simulink model "IntegrityControlModule"  (R2020b)
settings: Solver=VariableStepAuto  StartTime=0.0  StopTime=10.0  RelTol=1e-3
settings Model: Creator=leonk  LastModifiedBy=leonk

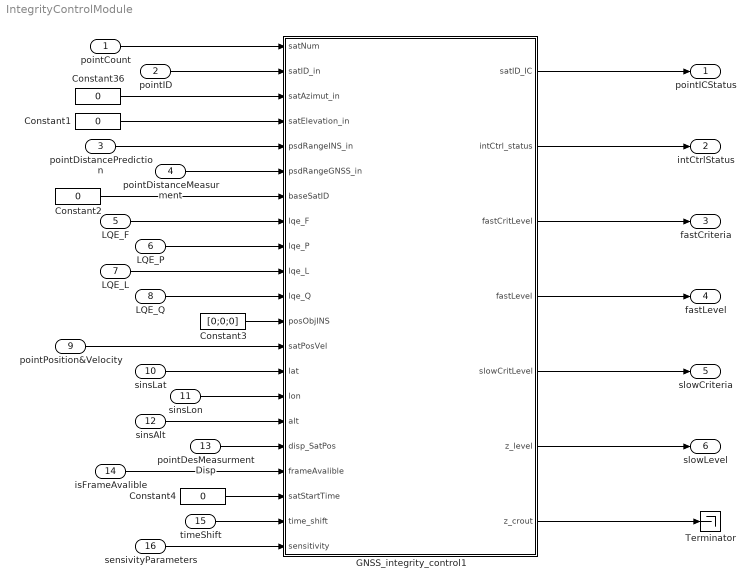
== system IntegrityControlModule ==
  pointCount : Inport  OutDataTypeStr=uint8
  pointID : Inport  Port=2
  pointDistancePrediction : Inport  Port=3  PortDimensions=[8,1]
  pointDistanceMeasurment : Inport  Port=4  PortDimensions=[8,1]
  LQE_F : Inport  Port=5
  LQE_P : Inport  Port=6
  LQE_L : Inport  Port=7
  LQE_Q : Inport  Port=8
  pointPosition&Velocity : Inport  Port=9  PortDimensions=[6,8]
  sinsLat : Inport  Port=10  PortDimensions=1
  sinsLon : Inport  Port=11  PortDimensions=1
  sinsAlt : Inport  Port=12  PortDimensions=1
  pointDesMeasurmentDisp : Inport  Port=13  PortDimensions=1
  isFrameAvalible : Inport  Port=14  OutDataTypeStr=uint8  PortDimensions=1
  timeShift : Inport  Port=15  PortDimensions=1
  sensivityParameters : Inport  Port=16  PortDimensions=[4,1]
  Constant{1..2,4,36} (4 alike) : Constant  Value=0
  Constant3 : Constant  Value=[0;0;0]
  GNSS_integrity_control1 : MATLAB Function  TreatAsAtomicUnit=on
  Terminator : Terminator
  pointICStatus : Outport  PortDimensions=32
  intCtrlStatus : Outport  Port=2  PortDimensions=32
  fastCriteria : Outport  Port=3
  fastLevel : Outport  Port=4  PortDimensions=32
  slowCriteria : Outport  Port=5  PortDimensions=32
  slowLevel : Outport  Port=6
  wires:
  pointCount/1 -> GNSS_integrity_control1/1(satNum)
  pointID/1 -> GNSS_integrity_control1/2(satID_in)
  Constant36/1 -> GNSS_integrity_control1/3(satAzimut_in)
  Constant1/1 -> GNSS_integrity_control1/4(satElevation_in)
  pointDistancePrediction/1 -> GNSS_integrity_control1/5(psdRangeINS_in)
  pointDistanceMeasurment/1 -> GNSS_integrity_control1/6(psdRangeGNSS_in)
  Constant2/1 -> GNSS_integrity_control1/7(baseSatID)
  LQE_F/1 -> GNSS_integrity_control1/8(lqe_F)
  LQE_P/1 -> GNSS_integrity_control1/9(lqe_P)
  LQE_L/1 -> GNSS_integrity_control1/10(lqe_L)
  LQE_Q/1 -> GNSS_integrity_control1/11(lqe_Q)
  Constant3/1 -> GNSS_integrity_control1/12(posObjINS)
  pointPosition&Velocity/1 -> GNSS_integrity_control1/13(satPosVel)
  sinsLat/1 -> GNSS_integrity_control1/14(lat)
  sinsLon/1 -> GNSS_integrity_control1/15(lon)
  sinsAlt/1 -> GNSS_integrity_control1/16(alt)
  isFrameAvalible/1 -> GNSS_integrity_control1/18(frameAvalible)
  Constant4/1 -> GNSS_integrity_control1/19(satStartTime)
  timeShift/1 -> GNSS_integrity_control1/20(time_shift)
  sensivityParameters/1 -> GNSS_integrity_control1/21(sensitivity)
  GNSS_integrity_control1/2(intCtrl_status) -> intCtrlStatus/1
  GNSS_integrity_control1/1(satID_IC) -> pointICStatus/1
  GNSS_integrity_control1/3(fastCritLevel) -> fastCriteria/1
  GNSS_integrity_control1/4(fastLevel) -> fastLevel/1
  GNSS_integrity_control1/5(slowCritLevel) -> slowCriteria/1
  GNSS_integrity_control1/6(z_level) -> slowLevel/1
  GNSS_integrity_control1/7(z_crout) -> Terminator/1
  pointDesMeasurmentDisp/1 -> GNSS_integrity_control1/17(disp_SatPos)

== matlab function IntegrityControlModule/GNSS_integrity_control1 ==
  data: satNum input uint8 size=1; satID_in input; satAzimut_in input; satElevation_in input; psdRangeINS_in input; psdRangeGNSS_in input; baseSatID input uint8 size=1; satID_IC output uint8; intCtrl_status output uint8 size=1; lqe_F input; lqe_P input; lqe_L input; lqe_Q input; posObjINS input size=3; satPosVel input; lat input; lon input; alt input; disp_SatPos input; frameAvalible input; fastCritLevel output; fastLevel output; slowCritLevel output; satStartTime input; time_shift input; sensitivity input size=[4,1]; z_level output; z_crout output

function [satID_IC, intCtrl_status, fastCritLevel, fastLevel, slowCritLevel,...
          z_level, z_crout]=  integrity_control(satNum, satID_in, satAzimut_in, satElevation_in, ...
                                                         psdRangeINS_in, psdRangeGNSS_in, baseSatID,...                                                     
                                                         lqe_F, lqe_P, lqe_L, lqe_Q, posObjINS, satPosVel, lat, lon, alt, disp_SatPos, frameAvalible, satStartTime, time_shift, sensitivity)

    persistent intCtrl qq time
%--------------------------------------------------------------------------
%Константы
    disp_SatVel = 0.03;
    
    
    
    if isempty(intCtrl)
               
        qq = 0;
        time = 0;
        slowWindow = 600;% set max for code generation
        satLimit   = 8;
        
%         intCtrl.sensitivity = zeros(3,1);
        intCtrl.slowSensitivity = sensitivity(3);
        
        intCtrl.fastInit = uint8(0);
        intCtrl.psdRangeFast = zeros(satLimit,3);
        intCtrl.fastSatList = zeros(satLimit,1);
        
        
        intCtrl.slowInit = uint8(0);
        intCtrl.psdRangeSlow = ones(slowWindow,satLimit);
        intCtrl.slowSatList  = zeros(satLimit,1);
        
        intCtrl.probSatID = uint8(zeros(satLimit,1));
        intCtrl.moniSatID = uint8(zeros(satLimit,1));
        
        intCtrl.probSatNum = uint8(0);
        intCtrl.moniSatNum = uint8(0);
        
        intCtrl.baseSatID = uint8(0);
        
        intCtrl.satLossFrame     = zeros(satLimit,2); %Строка 1 не задейстоввана?
        intCtrl.satLossFrameAlow = uint8(10);
        
        intCtrl.slowMean = zeros(satLimit,2);
        intCtrl.slowDisp = zeros(satLimit,1);
        
        intCtrl.fastExpt = zeros(satLimit,1);%Не задействовано
        
        intCtrl.fastExptCriteria = zeros(satLimit,2);
        
        intCtrl.criteriaScale = ones(2,1) .* [sensitivity(1); sensitivity(2)]; 
        
        intCtrl.slowWindow      = slowWindow;
        intCtrl.slowWindow_size = sensitivity(4);
        intCtrl.satLimit        = satLimit;
    end
%--------------------------------------------------------------------------
%Объявление выходых параметров 
    satID_IC       = uint8(zeros(8 ,1));%uint8(zeros(intCtrl.satLimit ,1));
    fastCritLevel  =       zeros(8,1);%zeros(intCtrl.satLimit ,1);
    fastLevel      =       zeros(8,1);%zeros(intCtrl.satLimit ,1);
    slowCritLevel  =       zeros(8,1);%zeros(intCtrl.satLimit ,1);
    intCtrl_status =       uint8(1); %%uint8(1); %
    z_crout        =       zeros(1,1);%zeros(1,1);
    z_level        =       zeros(8,1);%zeros(intCtrl.satLimit ,1);
    
%--------------------------------------------------------------------------
%Костыль для подержания много спутников (Если всегда +- 8 но подскакивает до 12)

    satID        = uint8(zeros(intCtrl.satLimit,1));
    satAzimut    =       zeros(intCtrl.satLimit,1);
    satElevation =       zeros(intCtrl.satLimit,1);
    psdRangeINS  =       zeros(intCtrl.satLimit,1);
    psdRangeGNSS =       zeros(intCtrl.satLimit,1);
    
    for ii = 1:satNum
        satID(ii)        = satID_in(ii);
        satAzimut(ii)    = satAzimut_in(ii);
        satElevation(ii) = satElevation_in(ii);
        psdRangeINS(ii)  = psdRangeINS_in(ii);
        psdRangeGNSS(ii) = psdRangeGNSS_in(ii);
    end

%--------------------------------------------------------------------------  
%Обновление ID базового спутника
    intCtrl.baseSatID = baseSatID;
%--------------------------------------------------------------------------
%Счетчик пропущенных измерений НКА. Для "рабочих" НКА, счетчик обнуляется 
    intCtrl.satLossFrame(:,2) = intCtrl.satLossFrame(:,2) + 1;
    for ii = 1:satNum
        if find(satID(ii) == intCtrl.satLossFrame(:,1))
            intCtrl.satLossFrame(ii,2) = 0;
        end
    end
%--------------------------------------------------------------------------
    if frameAvalible == 1                                                  %Ждать поступления измерения псевдодальности
                                                                           %Быстрый цикл  
%                                                                          Набор информации (первых и вторых разностей)
        intCtrl = fastCircle (intCtrl, satNum, satID, psdRangeGNSS, psdRangeINS, disp_SatPos,...
                              lqe_F, lqe_P, lqe_L, lqe_Q, lat, lon, alt, posObjINS, satPosVel, disp_SatVel);
                                                                            %Набор информации (первых разностей)
                                                                           %Проверка по критерию
        probSatCount = 0;
        %intCtrl.probSatID = uint8(zeros(intCtrl.satLimit,1));%
        intCtrl.probSatID = uint8(zeros(8,1));
        for ii = 1:satNum
            if abs(intCtrl.psdRangeFast(ii,3)) >= (intCtrl.fastExptCriteria(ii))
                probSatCount = probSatCount + 1;
                intCtrl.probSatID(probSatCount) = satID(ii);
            end
        end
                                                                            %Медленный цикл  
                                                                            %Набор информации (вторых разностей и среднего)
    intCtrl = slowCircleLogic(intCtrl, satNum, satID, psdRangeGNSS, psdRangeINS);
%     
    
    for ii = 1:satNum
        baseMean = 0;
        baseDisp = intCtrl.slowDisp(ii);
%         alpha = intCtrl.slowSensitivity;
%         Z = (intCtrl.slowMean(ii) -  baseMean) ./ sqrt(intCtrl.slowDisp(ii) * 2/intCtrl.slowWindow(1:intCtrl.slowWindow_size));
%may be ERROR        
        Z = (intCtrl.slowMean(ii) -  baseMean) ./ sqrt(intCtrl.slowDisp(ii) * 2/intCtrl.slowWindow_size);
%         Z_criteria = tinv(1 - intCtrl.slowSensitivity, intCtrl.slowWindow(1:intCtrl.slowWindow_size) - 2 - 1);
        Z_criteria = tinv(intCtrl.slowSensitivity, intCtrl.slowWindow_size - 2 - 1);%(1:intCtrl.slowWindow_size)
        z_level(ii) = abs(Z);
        z_crout = Z_criteria;
   %Slow circle decision-making segment
        if abs(Z) >= Z_criteria
            jj = find(satID(ii) == intCtrl.probSatID);
            if length(jj) == 0
                probSatCount = probSatCount + 1;        
                intCtrl.probSatID(probSatCount) = satID(ii);  
            end
        end
    end
    
    end
    
fastLevel     = abs(intCtrl.psdRangeFast(:,3));    
fastCritLevel = intCtrl.fastExptCriteria(:,1);
slowCritLevel = abs(intCtrl.slowMean(:,1));
% z_level = abs(Z);
% z_crout = Z_criteria;

%--------------------------------------------------------------------------
    
%--------------------------------------------------------------------------
                                                                            %Отбор спутников и формирование выходной информации
                                                                     
    id = 0;
    intCtrl_status = uint8(1);% 1 - IC pass; 0 - IC fault
    time = time + time_shift;
%     if time > (satStartTime + intCtrl.slowWindow(1:intCtrl.slowWindow_size) * 4) 
    if time > (satStartTime + intCtrl.slowWindow_size * 4)%(1:intCtrl.slowWindow_size)
        for ii = 1:satNum
            if find(satID(ii) == intCtrl.probSatID)
                id = id + 1;
                satID_IC(id) = satID(ii);
            end
        end
        if satNum - id <= 4  
            intCtrl_status = uint8(0);
        end
    end
    
end


%==========================================================================
function [D_rho, D_rho_dot] = fastCriteriaMath( a,e2,C,Ro_mark,R_tp,disp_SatPos_mem, ...
                                    ii,lat,lon,alt, psdRange,posObj, satPosVel,...
                                    disp_SatPos, disp_SatVel)
        
        
        dPsdRange_dLambda =  (1/psdRange(ii)) * (Ro_mark + alt)*cos(lat)*...
                                                (sin(lon)*(satPosVel(1,ii) - posObj(1)) - ...
                                                 cos(lon)*(satPosVel(2,ii) - posObj(2)));

        dPsdRange_dphi    =  (1/psdRange(ii))   * ...
                              ((satPosVel(1,ii) - posObj(1)) * (- cos(lon) * cos(lat) * R_tp + (Ro_mark + alt) * cos(lon) * sin(lat)) + ...%dRz_dLat
                               (satPosVel(2,ii) - posObj(2)) * (- sin(lon) * cos(lat) * R_tp + (Ro_mark + alt) * sin(lon) * sin(lat)) + ...%dRz_dLat
                               (satPosVel(3,ii) - posObj(3)) * (- (1 - e2) * sin(lat) * R_tp - ((1 - e2) * Ro_mark + alt) * cos(lat)));    %dRz_dLat

        dPsdVel_dot_dVe   =  (1/psdRange(ii)) * (...
                                sin(lon) * (satPosVel(1,ii) - posObj(1)) - ...
                                cos(lon) * (satPosVel(2,ii) - posObj(2)));

        dPsdVel_dot_dVn   =  (1/psdRange(ii)) * (...
                                cos(lon)*sin(lat)*(satPosVel(1,ii) - posObj(1)) + ...
                                sin(lon)*sin(lat)*(satPosVel(2,ii) - posObj(2)) - ...
                                cos(lat)*         (satPosVel(3,ii) - posObj(3)));

        dPsdRange_dAlt    = (-1/psdRange(ii))* (...
                                cos(lat)*cos(lon)*(satPosVel(1,ii) - posObj(1)) + ...
                                cos(lat)*sin(lon)*(satPosVel(2,ii) - posObj(2)) + ...
                                sin(lat)*         (satPosVel(3,ii) - posObj(3)));
%--------------------------------------------------------------------------
%Формирование дисперсий
        dPsdVel_dot_dVh   = (-1/psdRange(ii))* (...
                                cos(lon)*cos(lat)*(satPosVel(1,ii) - posObj(1)) + ...
                                sin(lon)*cos(lat)*(satPosVel(2,ii) - posObj(2)) + ...
                                sin(lat)*         (satPosVel(3,ii) - posObj(3)));
%--------------------------------------------------------------------------
%Пересчет из радиан в метры
                            
        ro_1 = a*(1-e2)/(1-e2*sin(lat)^2)^(3/2) + alt;
        ro_2 = a*(1-e2*sin(lat)^2)^(-1/2) + alt;                      
        dPsdRange_dLambda =  (1/(ro_2 * cos(lat))) * dPsdRange_dLambda;
        dPsdRange_dphi    =  (1/ro_1) * dPsdRange_dphi;                 
%--------------------------------------------------------------------------
        D_hor = sum(abs([dPsdRange_dLambda, dPsdRange_dphi ]) * [C(1,1), C(1,2) ;...
                                                            C(2,1), C(2,2)]);
        D_vel = sum(abs([dPsdVel_dot_dVe,   dPsdVel_dot_dVn]) * [C(3,3), C(3,4) ;...
                                                            C(4,3), C(4,4)]);    
                                                        
        D_alt  = abs(dPsdRange_dAlt)  * C(20,20);
        D_vAlt = abs(dPsdVel_dot_dVh) * C(21,21);


        D_rho     = D_hor + D_alt  + disp_SatPos + disp_SatPos_mem;
        D_rho_dot = D_vel + D_vAlt + 2*disp_SatVel;

end



function intCtrl = fastCircle(intCtrl, satNum, satID, psdRangeGNSS, psdRangeINS, disp_SatPos,...
                              lqe_F, lqe_P, lqe_L, lqe_Q, lat, lon, alt, posObjINS, satPosVel, disp_SatVel)
    
    persistent disp_SatPos_mem

    if isempty(disp_SatPos_mem)
        disp_SatPos_mem = zeros(size(disp_SatPos));
        disp_SatPos_mem = disp_SatPos;
    end

%--------------------------------------------------------------------------
%Константы    
    a = 6378136;
    e2 = 0.0066943662;
%--------------------------------------------------------------------------
%Матрица связи С (?)        
    C = lqe_F*lqe_P*lqe_F' + lqe_L*lqe_Q*lqe_L' + lqe_P + 2*lqe_F*lqe_P;
    Ro_mark = a / sqrt(1 - e2*(sin(lat))^2);
%--------------------------------------------------------------------------
%Коэффициенты (направляющие косинусы). Аналагично матрице связи Н (ЖСК)        
    
    dRz_dLat = a*e2*cos(lat)*sin(lat) / ((1 - e2*sin(lat)^2)^(3/2));
    R_tp     = sin(lat)*(a + alt) - cos(lat)*dRz_dLat;  

    if intCtrl.fastInit == 0
        for ii = 1:satNum
            intCtrl.psdRangeFast(ii, 1) = 1;%(psdRangeGNSS(ii) - psdRangeGNSS(intCtrl.baseSatID));
            intCtrl.psdRangeFast(ii, 2) = intCtrl.psdRangeFast(ii, 1);
            intCtrl.fastSatList(ii)     = satID(ii);
            intCtrl.fastInit            = uint8(1); 
        end
    end


    for ii = 1:satNum
        sID = find(satID(ii) == intCtrl.fastSatList);%Был ли этот спутник раньше
        if ~isempty(sID) %Если этот спутник уже есть и обрабатывается 
            
            thirdDifference_previous = intCtrl.psdRangeFast(sID, 1);
            intCtrl.psdRangeFast(sID, 1) = psdRangeGNSS(sID) - psdRangeINS(sID);
            intCtrl.psdRangeFast(sID, 3) = intCtrl.psdRangeFast(sID, 1) - thirdDifference_previous;                                               
%             
            [D_rho, D_rho_dot] = fastCriteriaMath( a,          e2,        C,  Ro_mark,      R_tp, disp_SatPos_mem(ii), ...
                                                  ii,      lat,      lon,       alt, psdRangeINS,   posObjINS, satPosVel, disp_SatPos(ii), disp_SatVel);
                                                  
            intCtrl.fastExptCriteria(sID,1) = intCtrl.criteriaScale(1) * sqrt(abs(D_rho)    );
            intCtrl.fastExptCriteria(sID,2) = intCtrl.criteriaScale(2) * sqrt(abs(D_rho_dot));
        
        else % Если появился спутник
            if ii <= intCtrl.satLimit % Если не превышен лимит н спутники
                if length(find(intCtrl.fastSatList == 0)) ~= 0% Если есть слоты для спутников
                    %------Инициализация
                    sID = find(intCtrl.fastSatList == 0, 1,'first');% Вязть первый пустой слот
                    intCtrl.fastSatList (sID)    = satID(ii);% Записать ID нового спутника
                    
                    %--------------------------------------
                    %Замена на 3 разности
                            thirdDifference_previous = intCtrl.psdRangeFast(sID, 1);
                            intCtrl.psdRangeFast(sID, 1) = psdRangeGNSS(sID) - psdRangeINS(sID);
                            intCtrl.psdRangeFast(sID, 3) = intCtrl.psdRangeFast(sID, 1) - thirdDifference_previous;  
                    
                  
                    [D_rho, D_rho_dot] = fastCriteriaMath(   a,          e2,        C, dRz_dLat,      R_tp, disp_SatPos_mem(ii), ...
                                                            ii,      lat,      lon,       alt, psdRangeINS,   posObjINS, satPosVel, disp_SatPos(ii), disp_SatVel);                           
                    intCtrl.fastExptCriteria(sID,1) = intCtrl.criteriaScale(1) * sqrt(abs(D_rho)    );
                    intCtrl.fastExptCriteria(sID,2) = intCtrl.criteriaScale(2) * sqrt(abs(D_rho_dot));
                    
                else % Если нет слотов
                    jj = find(intCtrl.satLossFrame(:,2) >= intCtrl.satLossFrameAlow, 1, 'first');%Найти просрочку
                    if ~isempty(jj)% Если есть просроченые спутники
                    %------Инициализация
                        intCtrl.fastSatList(jj)     = satID(ii);
                    %--------------------------------------
                    %Замена на 3 разности
                            thirdDifference_previous = intCtrl.psdRangeFast(sID, 1);
                            intCtrl.psdRangeFast(sID, 1) = psdRangeGNSS(sID) - psdRangeINS(sID);
                            intCtrl.psdRangeFast(sID, 3) = intCtrl.psdRangeFast(sID, 1) - thirdDifference_previous; 
                        
                                   
                        [D_rho, D_rho_dot] = fastCriteriaMath(	 a,          e2,        C, dRz_dLat,       R_tp, disp_SatPos_mem(ii), ...
                                                                ii,      lat,      lon,       alt, psdRangeINS,   posObjINS, satPosVel, disp_SatPos(ii), disp_SatVel);
                                                  
                        intCtrl.fastExptCriteria(sID,1) = intCtrl.criteriaScale(1) * sqrt(abs(D_rho)    );
                        intCtrl.fastExptCriteria(sID,2) = intCtrl.criteriaScale(2) * sqrt(abs(D_rho_dot));
                    end
                end
            end
        end
        
        
    end
    
end








function intCtrl = slowCircleLogic(intCtrl, satNum, satID, psdRangeGNSS, psdRangeINS)

%--------------------------------------------------------------------------
%Инициализация
    if intCtrl.slowInit == 0
        for ii = 1:satNum
            intCtrl.slowSatList(ii)    = satID(ii);
%             intCtrl.psdRangeSlow(:,ii) = intCtrl.psdRangeSlow(:,ii) .*...
%                 ((psdRangeGNSS(ii)                   - psdRangeINS(ii))     ...
%                - (psdRangeGNSS(intCtrl.baseSatID) - psdRangeINS(intCtrl.baseSatID)));
        end
        intCtrl.slowInit = uint8(1);
    end
%--------------------------------------------------------------------------
%Медленный цикл
    for ii = 1:satNum
%         if find(satID(ii) ~= intCtrl.probSatID)
        if find(satID(ii) == intCtrl.slowSatList) %Если спутник уже был
            intCtrl = slowCircleAction(intCtrl, ii, psdRangeGNSS(ii), psdRangeINS(ii)); %обработка
        else 
            if length(find(intCtrl.slowSatList == 0)) ~= 0% Если есть слоты для спутников
                %------Инициализация
                sID = find(intCtrl.slowSatList == 0, 1,'first');% Взять первый пустой слот
                intCtrl.slowSatList(sID) = satID(ii);
                %max set only here
                intCtrl.psdRangeSlow((1:intCtrl.slowWindow_size),sID) = ones(uint16(intCtrl.slowWindow_size),1).*...
                                                 (psdRangeGNSS(ii)                - psdRangeINS(ii));% - ...
                                                  %(psdRangeGNSS(intCtrl.baseSatID) - psdRangeINS(intCtrl.baseSatID)));
                intCtrl = slowCircleAction(intCtrl, sID, psdRangeGNSS(ii), psdRangeINS(ii));
                fkngtest = 1;
            else % Если нет слотов
                jj = find(intCtrl.satLossFrame(:,2) >= intCtrl.satLossFrameAlow, 1, 'first');%Найти просрочку
                if ~isempty(jj)% Если есть просроченые спутники
                %------Инициализация
                    intCtrl.slowSatList(jj) = satID(ii);
                    intCtrl.psdRangeSlow((1:intCtrl.slowWindow_size),jj) = ones(uint16(intCtrl.slowWindow_size),1).*...
                                                    (psdRangeGNSS(ii)                - psdRangeINS(ii));
                    intCtrl = slowCircleAction(intCtrl, jj, psdRangeGNSS(ii), psdRangeINS(ii));
                end
            end
        end
            
            
            
            
            
%             if ii <= intCtrl.satLimit %Если не превышено количество спутников
%                 jj = find(intCtrl.satLossFrame(:,2) >= intCtrl.satLossFrameAlow, 1, 'first');% 
%                 intCtrl.slowSatList(jj) = satID(ii);
% 
%                 intCtrl.psdRangeSlow(:,jj) = ones(intCtrl.slowWindow(1:slowWindow_size),1).*...
%                                                 ((psdRangeGNSS(ii)                - psdRangeINS(ii))...
%                                                - (psdRangeGNSS(intCtrl.baseSatID) - psdRangeINS(intCtrl.baseSatID)));
% 
%                 intCtrl = slowCircleAction(intCtrl, jj, psdRangeGNSS, psdRangeINS);
%             end
%         end
%         end
    end
end

function intCtrl = slowCircleAction(intCtrl, id, psdRangeGNSS, psdRangeINS)

    intCtrl.psdRangeSlow(1:intCtrl.slowWindow_size,id) = circshift(intCtrl.psdRangeSlow(1:intCtrl.slowWindow_size,id),1);
    intCtrl.psdRangeSlow(1,id) = (psdRangeGNSS - psdRangeINS);
   %intCtrl.psdRangeSlow(1,id) = (psdRangeGNSS(id) - psdRangeINS(id)) - (psdRangeGNSS(intCtrl.baseSatID) - psdRangeINS(intCtrl.baseSatID));  
    intCtrl.psdRangeSlow(1,id) = intCtrl.psdRangeSlow(1,id) - intCtrl.slowMean(id,2);
    intCtrl.slowMean(id,2)     = (psdRangeGNSS - psdRangeINS);
    
    
    intCtrl.slowMean(id,1)= mean(intCtrl.psdRangeSlow(1:intCtrl.slowWindow_size,id));
    intCtrl.slowDisp(id)  =  std(intCtrl.psdRangeSlow(1:intCtrl.slowWindow_size,id));
end
